simulink model "sim_lab3_recapitulare"  (R2024b)
settings: Solver=VariableStepAuto  StartTime=0.0  StopTime=10.0  RelTol=1e-3
values from neighbouring files (symbols this model uses):
  A = [-1, 0, 0; -1 -2 -101; 1, 1, 0;]    [Lab3.m]    (also in Lab3_recapitulare.m = [-1, 0, 0; -1, -2, 101; 1, 1, 0])
  b = [0; 1; 0;]    [Lab3.m]    (also in Lab3_recapitulare.m = [0; 1; 0])
  c_T = [1, 0, 101]    [Lab3.m]    (also in Lab3_recapitulare.m)
  D = 0    [Lab3.m]    (also in Lab3_recapitulare.m)
libraries: simulink x2
settings Model: Creator=akopo  LastModifiedBy=akopo

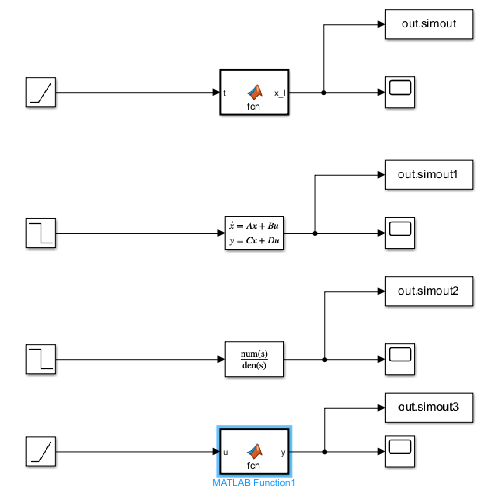
[thumbnail: Simulink's stored preview of the top-level diagram]
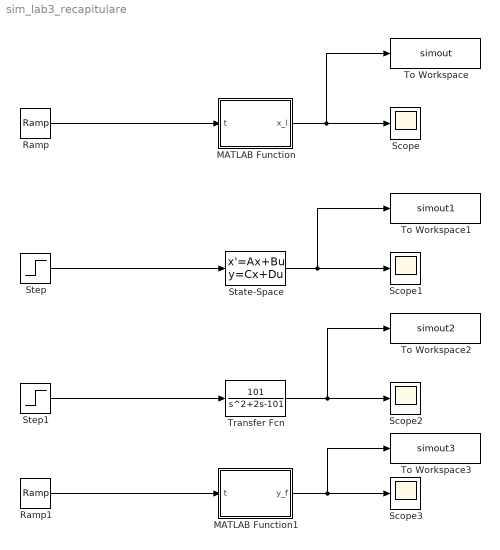
== system sim_lab3_recapitulare ==
  MATLAB Function : MATLAB Function  TreatAsAtomicUnit=on
  MATLAB Function1 : MATLAB Function  TreatAsAtomicUnit=on
  Ramp : simulink/Sources/Ramp  slope=1  start=0  InitialOutput=0
  Ramp1 : simulink/Sources/Ramp  slope=1  start=0  InitialOutput=0
  Scope{,1..3} (4 alike) : Scope
  State-Space : StateSpace  A=A  B=b  C=c_T  D=D  InitialCondition=0
  Step : Step  Time=0  After=-2  SampleTime=0
  Step1 : Step  Time=0  After=-2  SampleTime=0
  To Workspace : ToWorkspace  VariableName=simout  SaveFormat=Timeseries  SampleTime=-1
  To Workspace1 : ToWorkspace  VariableName=simout1  SaveFormat=Timeseries  SampleTime=-1
  To Workspace2 : ToWorkspace  VariableName=simout2  SaveFormat=Timeseries  SampleTime=-1
  To Workspace3 : ToWorkspace  VariableName=simout3  SaveFormat=Timeseries  SampleTime=-1
  Transfer Fcn : TransferFcn  Numerator=[101]  Denominator=[1 2 -101]
  wires:
  MATLAB Function/1(x_l) -> To Workspace/1, Scope/1
  Ramp/1 -> MATLAB Function/1(t)
  Step/1 -> State-Space/1
  State-Space/1 -> To Workspace1/1, Scope1/1
  Step1/1 -> Transfer Fcn/1
  Transfer Fcn/1 -> To Workspace2/1, Scope2/1
  Ramp1/1 -> MATLAB Function1/1(t)
  MATLAB Function1/1(y_f) -> To Workspace3/1, Scope3/1

== matlab function sim_lab3_recapitulare/MATLAB Function ==
  data: t input; x_l output
function x_l = fcn(t)

x_l = [exp(-t), exp(-t)*(cos(10*t) - sin(10*t)/10) - exp(-t) + (101*sin(10*t)*exp(-t))/10, (sin(10*t)*exp(-t))/10 - exp(-t)*(cos(10*t) + sin(10*t)/10)];

== matlab function sim_lab3_recapitulare/MATLAB Function1 ==
  data: t input; y_f output
function y_f = fcn(t)

y_f = 2*exp(-t)*(cos(10*t) + sin(10*t)/10) - 2;
